simulink model "deployAMR_stateflow"  (R2024a)
settings: configuration reference "SharedConfig" (kept outside this file)
model workspace (MAT data in the model file):
  mdlWSDbList : string (value not decoded)
  mdlWSDbcList : string (value not decoded)
undefined symbols (not defined in the file): L, L_limited, magnitude, max_steering_angle_deg, num_of_wps, T, tstep, vehicle_wheelbase
libraries: simulink x3, simulink_extras x2
(part 2 of 2)

== system deployAMR_stateflow/Trajectory_module1/Trajectory_controller_moving/long_deg2meters_2 ==
  source_lat : Inport
  destination_lat : Inport  Port=2
  Add : Sum  Inputs=+-
  range_meters : Outport
  wires:
  Add/1 -> range_meters/1
  destination_lat/1 -> Add/1
  source_lat/1 -> Add/2

== system deployAMR_stateflow/Trajectory_module1/Trajectory_controller_moving/long_deg2meters_4 ==
  source_lon : Inport
  destination_lon : Inport  Port=2
  Add1 : Sum  Inputs=+-
  range_meters : Outport
  wires:
  source_lon/1 -> Add1/2
  Add1/1 -> range_meters/1
  destination_lon/1 -> Add1/1

== system deployAMR_stateflow/Trajectory_module1/Trajectory_controller_moving/long_deg2meters_5 ==
  source_lon : Inport
  destination_lon : Inport  Port=2
  Add : Sum  Inputs=+-
  range_meters : Outport
  wires:
  source_lon/1 -> Add/2
  destination_lon/1 -> Add/1
  Add/1 -> range_meters/1

== system deployAMR_stateflow/Trajectory_module1/Trajectory_controller_moving/long_deg2meters_6 ==
  source_lon : Inport
  destination_lon : Inport  Port=2
  Add : Sum  Inputs=+-
  range_meters : Outport
  wires:
  Add/1 -> range_meters/1
  destination_lon/1 -> Add/1
  source_lon/1 -> Add/2

== system deployAMR_stateflow/Trajectory_module1/Waypoint_Selector/distance_1 ==
  dx_meters : Inport
  dy_meters : Inport  Port=2
  Add : Sum
  Divide1 : Product  Inputs=**
  Divide2 : Product  Inputs=**
  Sqrt : Sqrt
  distance_meters : Outport
  wires:
  dx_meters/1 -> Divide1/2, Divide1/1
  Divide1/1 -> Add/1
  Add/1 -> Sqrt/1
  dy_meters/1 -> Divide2/2, Divide2/1
  Divide2/1 -> Add/2
  Sqrt/1 -> distance_meters/1

== system deployAMR_stateflow/Trajectory_module1/Waypoint_Selector/lat_deg2meters_3 ==
  source_lat : Inport
  dest_lat : Inport  Port=2
  Add : Sum  Inputs=+-
  range_meters : Outport
  wires:
  Add/1 -> range_meters/1
  dest_lat/1 -> Add/1
  source_lat/1 -> Add/2

== system deployAMR_stateflow/Trajectory_module1/Waypoint_Selector/long_deg2meters_3 ==
  source_lon : Inport
  dest_lon : Inport  Port=2
  Add1 : Sum  Inputs=+-
  range_meters1 : Outport
  wires:
  source_lon/1 -> Add1/2
  dest_lon/1 -> Add1/1
  Add1/1 -> range_meters1/1

== matlab function deployAMR_stateflow/Backup/GPS_speed_measure/MATLAB Function ==
  data: lat1 input; theta output; lat2 input; lon1 input; lon2 input
function theta = angle(lat1, lat2, lon1, lon2)
    lat2 = lat2 * pi/180;
    lat1 = lat1 * pi/180;
    lon1 = lon1 * pi/180;
    lon2 = lon2 * pi/180;
    
    t1 = tan( lat2/2 + pi/4 );
    t2 = tan( lat1/2 + pi/4);
    dphi = log(t1/t2);
    dlon = abs(lon1-lon2);
    theta = atan2( mod(dlon, 180) , dphi)*180/pi;

== stateflow chart deployAMR_stateflow/AMR_stateFlow ==
  state S0_startup
    entry:
    %to_web("AGV entered boot mode (S0_startup)");
    state = 0;
    moving = 0;
    settings: description=This state models the modes of a window sensor and implements logic to respond when that sensor is producing a signal.
  state E1_failed
    entry:
    state = -1;
    moving = 0;
    %to_web("AGV failed to startup (E1_failed)!");
    settings: description=This state models the modes of a window sensor and implements logic to respond when that sensor is producing a signal.
  state autonomousOperation
    settings: description=This state models the modes of a window sensor and implements logic to respond when that sensor is producing a signal.
    state S2_engaged
      entry:
      %to_web("AGV is engaged mode (S2_engaged)");
      state = 2;
      settings: description=This state models the modes of a window sensor and implements logic to respond when that sensor is producing a signal.
      state S2A_Init
        entry:
        %to_web("AGV is rotating (S2A_Init)")
        moving = 0;
      state S2B_Moving
        entry:
        %to_web("AGV is moving (S2B_Moving)")
        moving = 1;
      state S2C_Parking
        entry:
        %to_web("AGV is slowing down (S2C_Parking)")
        moving = 2;
      state S2D_Stopped
        entry:
        %to_web("AGV is stopped (S2D_Stopped)")
        moving = 0;
      state S2E_Gate
        entry:
        %to_web("AGV is waiting gate Open (S2E_Gate)");
        moving = 0;
      (default) -> S2A_Init
      S2B_Moving -> (junction 285) [order 1] : [AMR_near_impact==TRUE]
      (junction 285) -> (junction 290)
      S2A_Init -> S2B_Moving : [AMR_alpha_angle <= 30]
      S2B_Moving -> S2C_Parking [order 2] : [AMR_alpha_angle >= 60| AMR_closedGate_ahead==TRUE | AMR_inDestination==TRUE]
      (junction 300) -> S2A_Init
      S2C_Parking -> (junction 290) [order 1] : [AMR_near_impact==TRUE]
      (junction 290) -> (junction 286)
      (junction 299) -> (junction 300)
      S2E_Gate -> (junction 300) [order 2] : [AMR_closedGate_ahead==TRUE]
      (junction 295) -> (junction 299) [order 3]
      S2C_Parking -> S2D_Stopped [order 2] : [AMR_measured_speed < 0.015]
      S2E_Gate -> S2E_Gate [order 1] : after(60, sec)
      (junction 295) -> S2E_Gate [order 2] : [AMR_closedGate_ahead==TRUE]
      S2D_Stopped -> (junction 295) : [AMR_near_impact==FALSE && AMR_measured_speed < 0.015]
      (junction 286) -> S2D_Stopped : %{to_web("AGV is near impact!");}
    state S1_standby
      entry:
      %to_web("AGV is waiting instructions (S1_standby)");
      state = 1;
      settings: description=This state models the modes of a window sensor and implements logic to respond when that sensor is producing a signal.
    state S4_unloading [commented out]
      entry:
      %to_web("AGV starting unloading process");
      state = 4;
      settings: description=This state models the modes of a window sensor and implements logic to respond when that sensor is producing a signal.
    state S3_loading [commented out]
      entry:
      %to_web("AGV starting loading process");
      state = 3;
      settings: description=This state models the modes of a window sensor and implements logic to respond when that sensor is producing a signal.
    (default) -> S1_standby
    S1_standby -> S2_engaged : [AMR_routeDefined==TRUE]
    S4_unloading -> S1_standby [commented out]
    (junction 269) -> S2_engaged [commented out]
    S3_loading -> (junction 269) [commented out]
    (junction 295) -> (junction 253) [order 1] : [AMR_inDestination==TRUE]
    (junction 333) -> S2D_Stopped
    (junction 275) -> S4_unloading [commented out]
    (junction 254) -> S3_loading [commented out] : [AGV_withLoad==FALSE]
    (junction 254) -> (junction 275) : [AMR_withLoad==TRUE]
    (junction 253) -> (junction 254) [order 1]
    (junction 253) -> (junction 333) [order 2]
  note: Constantes:
      | WAITING = 0
      | SUCCESS=1
      | FAIL=-1
      | FALSE=0
      | TRUE=1
      |
      | Flags:
      | AGV_speed_measued = double() => Captura a velocidade do AGV
      | AGV_target_angle = double() => Captura o ângulo entre o AGV e o próximo waypoing
      | AGV_near_impact = TRUE => Sensor acusa impacto iminente
      | AGV_near_impact = FALSE => Sensor de impacto diz que está livre
      | AGV_ext_safety_plc = TRUE => Estado de emergência foi resolvido
      | AGV_ext_safety_plc = FALSE => Estado de emergência não foi resolvido
      | AGV_closedGate_ahead = TRUE => Existe um portão fechado a frente
      | AGV_closedGate_ahead = FALSE => Caminho livre
      | AGV_withLoad = TRUE => AGV está com carga (segue para estado de unloading)
      | AGV_withLoad = FALSE => AGV está sem carga (segue para o estado de loading)
      | AGV_inDestination = TRUE => AGV chegou ao destino de carga ou descarga
      | AGV_inDestination = FAIL => AGV chegou ao destino de carga ou descarga
      | AGV_system_startup = WAITING => AGV não foi inicializado (aguardando)
      | AGV_system_startup = SUCCESS => AGV inicializado com sucesso
      | AGV_system_startup = FAIL => AGV inicializado com falha
      | AGV_system_emergency = TRUE => AGV vai para modo de emergência
      | AGV_system_emergency = FALSE => AGV continua sua operação normal
      | AGV_manual_mode = TRUE => AGV vai para modo manual
      | AGV_manual_mode = FALSE => AGV continua sua operação normal
      | AGV_routeDefined = TRUE => AGV com rota definida
      | AGV_routeDefined = FALSE => AGV sem rota definida
  state E2_emergency
    entry:
    state = -2;
    moving = 0;
    %fprintf("AGV está em modo de emergência!");
    settings: description=This state models the modes of a window sensor and implements logic to respond when that sensor is producing a signal.
  state E3_manualMode
    entry:
    state = -3;
    moving = 0;
    %fprintf("to web: AGV está em modo manual!\n");
    settings: description=This state models the modes of a window sensor and implements logic to respond when that sensor is producing a signal.
  (default) -> (junction 244)
  (junction 242) -> (junction 244)
  (junction 244) -> S0_startup
  (junction 312) -> (junction 242)
  S0_startup -> (junction 257) : [AMR_system_start~=WAITING]
  (junction 257) -> (junction 251) [order 1] : [AMR_system_start==FAIL]
  (junction 251) -> E1_failed
  (junction 257) -> autonomousOperation [order 2] : [AMR_system_start==SUCCESS]
  autonomousOperation -> E1_failed [order 3] : [AMR_system_start==FAIL]
  E1_failed -> (junction 312)
  (junction 243) -> (junction 312)
  E2_emergency -> (junction 243) [order 1] : [AMR_ext_safety_plc==TRUE]
  autonomousOperation -> E2_emergency [order 1] : [AMR_set_emergency==TRUE]
  E2_emergency -> E2_emergency [order 2] : after(10, sec)
  autonomousOperation -> E3_manualMode [order 2] : [AMR_manual_mode==TRUE | AMR_idle_mode==TRUE]
  E3_manualMode -> autonomousOperation : [AMR_manual_mode==FALSE | AMR_idle_mode==FALSE]
  data: msg function_input; state output =0; moving output size=1; FAIL constant double =-1; SUCCESS constant double =1; WAITING constant double =0; AMR_closedGate_ahead input; AMR_ext_safety_plc input; AMR_inDestination input; AMR_manual_mode input; AMR_idle_mode input; AMR_measured_speed input; AMR_near_impact input; AMR_set_emergency input; AMR_system_start input; AMR_alpha_angle input; AMR_withLoad input; FALSE constant double =0; TRUE constant double =1; AMR_routeDefined input
  function to_web(msg):
    | % Envia um log para o servidor local (em python)
    | function to_web(msg)
    |     fprintf("to web: %s\n",msg);
    |     udps = dsp.UDPSender('RemoteIPPort',31000);
    |     udps(uint8(char(msg)))
    |     release(udps)
